simulink model "lab1_ea"  (Simulink 8.5)
settings: Solver=ode45  StartTime=0.0  StopTime=10.0  RelTol=1e-3
libraries: simulink x2
settings Model: Creator=Tabi  LastModifiedBy=Tabi
settings DataIOCC: SignalLoggingSaveFormat=Dataset
settings OptimizationCC: ExpressionDepthLimit=128
settings DebuggingCC: UnderspecifiedInitializationDetection=Simplified  MergeDetectMultiDrivingBlocksExec=error  FcnCallInpInsideContextMsg=EnableAllAsError  StateNameClashWarn=none
settings GRTTargetCC: CombineOutputUpdateFcns=on  GRTInterface=off

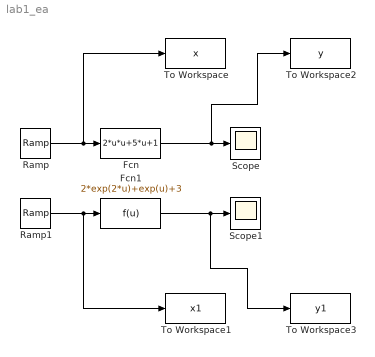
== system lab1_ea ==
  Fcn : Fcn  Expr=2*u*u+5*u+1
  Fcn1 : Fcn  Expr=2*exp(2*u)+exp(u)+3
  Ramp : simulink/Sources/Ramp  slope=1  start=0  X0=-3
  Ramp1 : simulink/Sources/Ramp  slope=1  start=0  X0=-3
  Scope : Scope
  Scope1 : Scope
  To Workspace : ToWorkspace  VariableName=x  SaveFormat=Timeseries  SampleTime=-1
  To Workspace1 : ToWorkspace  VariableName=x1  SaveFormat=Timeseries  SampleTime=-1
  To Workspace2 : ToWorkspace  VariableName=y  SaveFormat=Timeseries  SampleTime=-1
  To Workspace3 : ToWorkspace  VariableName=y1  SaveFormat=Timeseries  SampleTime=-1
  wires:
  Ramp/1 -> To Workspace/1, Fcn/1
  Fcn/1 -> To Workspace2/1, Scope/1
  Ramp1/1 -> To Workspace1/1, Fcn1/1
  Fcn1/1 -> To Workspace3/1, Scope1/1
